simulink model "noise"  (R2017b)
settings: Solver=FixedStepAuto  StartTime=0.0  StopTime=100  FixedStep=0.01  MaxStep=0.01  RelTol=1e-3
values from neighbouring files (symbols this model uses):
  b1 = 1    [test.m]
  b2 = 2    [test.m]
libraries: simulink x1
settings Model: Creator=rablanco.ext  LastModifiedBy=rablanco.ext

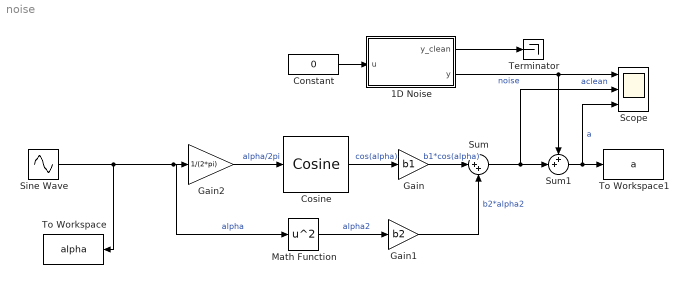
== system noise ==
  1D Noise : MATLAB Function  TreatAsAtomicUnit=on
  Constant : Constant  Value=0
  Cosine : simulink/Lookup Tables/Cosine  Formula=cos(2*pi*u)  NumDataPoints=(2^8)+1  OutputWordLength=16  InternalRulePriority=Speed
      settings: SourceProductName=Simulink  SourceProductBaseCode=SL
  Gain : Gain  Gain=b1
  Gain1 : Gain  Gain=b2
  Gain2 : Gain  Gain=1/(2*pi)
  Math Function : Math  Operator=square  SaturateOnIntegerOverflow=on
  Scope : Scope  NumInputPorts=3
  Sine Wave : Sin  SampleTime=0
  Sum : Sum  Inputs=|++
  Sum1 : Sum  Inputs=++|
  Terminator : Terminator
  To Workspace : ToWorkspace  VariableName=alpha  SampleTime=-1
  To Workspace1 : ToWorkspace  VariableName=a  SampleTime=-1
  wires:
  1D Noise/1(y_clean) -> Terminator/1
  1D Noise/2(y) -> Sum1/1, Scope/1  "noise"
  Sine Wave/1 -> Math Function/1, Gain2/1, To Workspace/1  "alpha"
  Cosine/1 -> Gain/1  "cos(alpha)"
  Math Function/1 -> Gain1/1  "alpha2"
  Gain/1 -> Sum/1  "b1*cos(alpha)"
  Gain1/1 -> Sum/2  "b2*alpha2"
  Sum/1 -> Sum1/2, Scope/2  "aclean"
  Gain2/1 -> Cosine/1  "alpha/2pi"
  Constant/1 -> 1D Noise/1(u)
  Sum1/1 -> Scope/3, To Workspace1/1  "a"

== matlab function noise/1D Noise ==
  data: y_clean output; u input; y output
function [y_clean,y] = fcn(u)
y_clean = u;
max_u=1;
noise = max_u.*1.*(-1+2.*rand(1)); % rand num (-1,1)*(25% of u)->(-25%,25%) of u
y = u+ noise;
